simulink model "simulation_pid_controller"  (R2019a)
settings: Solver=FixedStepAuto  StartTime=0.0  StopTime=0.5  FixedStep=0.001  RelTol=1e-3
undefined symbols (not defined in the file or in its folder): rho
libraries: simulink x1
settings Model: Creator=user  LastModifiedBy=user

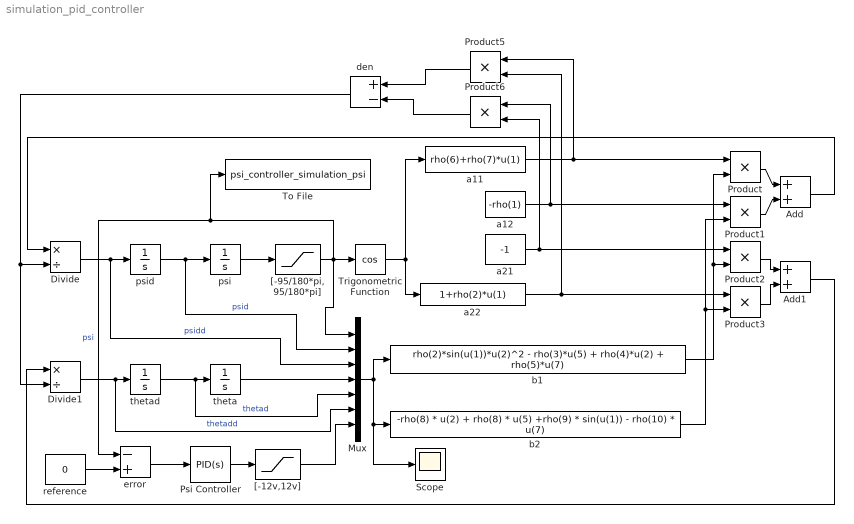
== system simulation_pid_controller ==
  Add : Sum
  Add1 : Sum
  Divide : Product  Inputs=*/
  Divide1 : Product  Inputs=*/
  Mux : Mux  Inputs=7
  Product{,1..3,5..6} (6 alike) : Product
  Psi Controller : simulink/Continuous/PID Controller  Controller=PID  Form=Parallel  TimeDomain=Continuous-time  SampleTime=-1  IntegratorMethod=Forward Euler  FilterMethod=Forward Euler  ControllerParametersSource=internal  P=95.3  I=600  D=1.1  UseFilter=on  N=1000  TunerSelectOption=Transfer Function Based (PID Tuner App)  InitialConditionSource=internal  InitialConditionForIntegrator=0  InitialConditionForFilter=0  DifferentiatorICPrevScaledInput=0  ExternalReset=none  TrackingMode=off  Kt=1  LimitOutput=off  UpperSaturationLimit=inf  LowerSaturationLimit=-inf  LinearizeAsGain=on  AntiWindupMode=none  Kb=1  POutMin=[]  POutMax=[]  IOutMin=[]  IOutMax=[]  DOutMin=[]  DOutMax=[]  NOutMin=[]  NOutMax=[]  SumOutMin=[]  SumOutMax=[]  SaturationOutMin=[]  SaturationOutMax=[]  PParamMin=[]  PParamMax=[]  IParamMin=[]  IParamMax=[]  DParamMin=[]  DParamMax=[]  NParamMin=[]  NParamMax=[]  KbParamMin=[]  KbParamMax=[]  KtParamMin=[]  KtParamMax=[]  KbOutMin=[]  KbOutMax=[]  KtOutMin=[]  KtOutMax=[]  IntegratorOutMin=[]  IntegratorOutMax=[]  FilterOutMin=[]  FilterOutMax=[]  SumI1OutMin=[]  SumI1OutMax=[]  SumI2OutMin=[]  SumI2OutMax=[]  SumI3OutMin=[]  SumI3OutMax=[]  SumI4OutMin=[]  SumI4OutMax=[]  SumDOutMin=[]  SumDOutMax=[]  DifferentiatorOutMin=[]  DifferentiatorOutMax=[]  FilterDiffOutCoefMin=[]  FilterDiffOutCoefMax=[]  ReciprocalOutMin=[]  ReciprocalOutMax=[]  SumDenOutMin=[]  SumDenOutMax=[]  SumNumOutMin=[]  SumNumOutMax=[]  DivideOutMin=[]  DivideOutMax=[]  IntegratorContinuousStateAttributes=''  IntegratorStateMustResolveToSignalObject=off  IntegratorRTWStateStorageClass=Auto  FilterContinuousStateAttributes=''  FilterStateMustResolveToSignalObject=off  FilterRTWStateStorageClass=Auto  ParallelPVariant=InternalParameters  IdealPVariant=Disabled  IVariant=InternalParameters  DVariant=InternalParameters  IntegratorVariant=Continuous  SatVariant=Disabled  AWVariant=Passthrough  PCopyVariant=Disabled  TRVariant=Disabled  FdbkBlocksVariant=Forward  IdealPFdbkVariant=Disabled  SatFdbkVariant=Disabled  DerivativeFilterVariant=ContFilter  NVariant=InternalParameters  NCopyVariant=Disabled  FilterICVariant=InternalICsFilter  IntegratorICVariant=InternalICs  ExternalResetVariant=Disabled  TRSumVariant=Passthrough  SumFdbkVariant=Disabled  SumVariant=Sum_PID
  Scope : Scope
  To File : ToFile  Filename=psi_controller_simulation_psi  MatrixName=psi  SaveFormat=Timeseries
  Trigonometric Function : Trigonometry  Operator=cos
  "[-12v,12v]" : Saturate  UpperLimit=12  LowerLimit=-12
  "[-95/180*pi, 95/180*pi]" : Saturate  UpperLimit=95/180*pi  LowerLimit=-95/180*pi
  a11 : Fcn  Expr=rho(6)+rho(7)*u(1)
  a12 : Constant  Value=-rho(1)
  a21 : Constant  Value=-1
  a22 : Fcn  Expr=1+rho(2)*u(1)
  b1 : Fcn  Expr=rho(2)*sin(u(1))*u(2)^2 - rho(3)*u(5) + rho(4)*u(2) + rho(5)*u(7)
  b2 : Fcn  Expr=-rho(8) * u(2) + rho(8) * u(5) +rho(9) * sin(u(1)) - rho(10) * u(7)
  den : Sum  Inputs=+-
  error : Sum  Inputs=-+
  psi : Integrator  InitialCondition=0.05
  psid : Integrator
  reference : Constant  Value=0
  theta : Integrator
  thetad : Integrator
  wires:
  psid/1 -> psi/1, Mux/2  "psid"
  thetad/1 -> Mux/5, theta/1  "thetad"
  Divide/1 -> Mux/3, psid/1  "psidd"
  Divide1/1 -> Mux/6, thetad/1  "thetadd"
  psi/1 -> "[-95/180*pi, 95/180*pi]"/1
  "[-95/180*pi, 95/180*pi]"/1 -> To File/1, error/1, Mux/1, Trigonometric Function/1  "psi"
  Trigonometric Function/1 -> a11/1, a22/1
  a11/1 -> Product5/1, Product/1
  a12/1 -> Product6/1, Product1/1
  b1/1 -> Product2/2, Product/2
  b2/1 -> Product3/2, Product1/2
  a21/1 -> Product6/2, Product2/1
  a22/1 -> Product5/2, Product3/1
  Product/1 -> Add/1
  Product1/1 -> Add/2
  Product2/1 -> Add1/1
  Product3/1 -> Add1/2
  Add/1 -> Divide/1
  Add1/1 -> Divide1/1
  Product5/1 -> den/1
  Product6/1 -> den/2
  den/1 -> Divide/2, Divide1/2
  theta/1 -> Mux/4
  error/1 -> Psi Controller/1
  reference/1 -> error/2
  "[-12v,12v]"/1 -> Mux/7
  Psi Controller/1 -> "[-12v,12v]"/1
  Mux/1 -> b1/1, Scope/1, b2/1
